simulink model "simulink_mecha_base"  (R2016b)
settings: Solver=VariableStepAuto  StartTime=0.0  StopTime=50  RelTol=1e-3
libraries: simulink x1
settings Model: Creator=Utente  LastModifiedBy=Utente

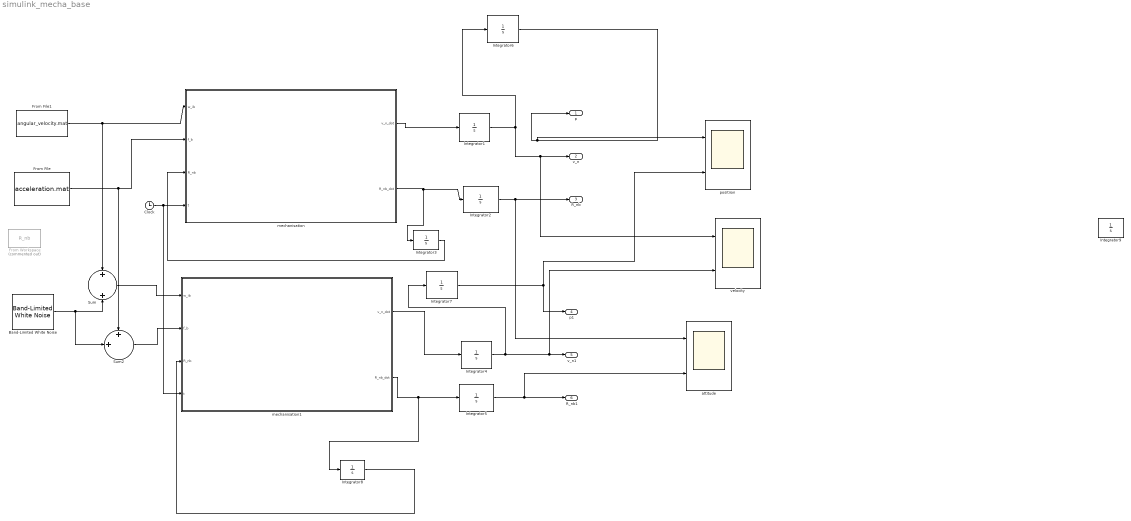
== system simulink_mecha_base ==
  Band-Limited White Noise : simulink/Sources/Band-Limited White Noise  Cov=[100 100 100]  Ts=0.1  seed=[23341]  VectorParams1D=off
  Clock : Clock
  From Workspace : FromWorkspace  Commented=on  VariableName=R_nb  SampleTime=0
  From File : FromFile  FileName=acceleration.mat  SampleTime=0
  From File1 : FromFile  FileName=angular_velocity.mat  SampleTime=0
  Integrator{1..9} (9 alike) : Integrator
  Sum : Sum  Inputs=+|+
  Sum2 : Sum  Inputs=++|
  attitude : Scope  NumInputPorts=2
  mechanisation : MATLAB Function  TreatAsAtomicUnit=on
  mechanisation1 : MATLAB Function  TreatAsAtomicUnit=on
  positiion : Scope  NumInputPorts=2
  velocity : Scope  NumInputPorts=2
  " p" : Outport
  " v_n" : Outport  Port=2
  " R_nb" : Outport  Port=3
  " p1" : Outport  Port=4
  " v_n1" : Outport  Port=5
  " R_nb1" : Outport  Port=6
  wires:
  mechanisation/1(v_n_dot) -> Integrator1/1
  Integrator1/1 -> velocity/1, " v_n"/1, Integrator6/1
  Integrator2/1 -> attitude/1, " R_nb"/1
  mechanisation1/1(v_n_dot) -> Integrator4/1
  Integrator7/1 -> " p1"/1, positiion/2
  Integrator4/1 -> Integrator7/1, velocity/2, " v_n1"/1
  Integrator5/1 -> attitude/2, " R_nb1"/1
  From File/1 -> mechanisation/2(f_b), Sum2/1
  From File1/1 -> Sum/1, mechanisation/1(w_ib)
  Band-Limited White Noise/1 -> Sum2/2, Sum/2
  Sum/1 -> mechanisation1/1(w_ib)
  Sum2/1 -> mechanisation1/2(f_b)
  Integrator6/1 -> " p"/1, positiion/1
  mechanisation/2(R_nb_dot) -> Integrator3/1, Integrator2/1
  Integrator3/1 -> mechanisation/3(R_nb)
  Clock/1 -> mechanisation1/4(t), mechanisation/4(t)
  Integrator8/1 -> mechanisation1/3(R_nb)
  mechanisation1/2(R_nb_dot) -> Integrator8/1, Integrator5/1

== matlab function simulink_mecha_base/mechanisation1 ==
  data: w_ib input; f_b input; v_n_dot output; R_nb_dot output; R_nb input; t input
function [v_n_dot, R_nb_dot] = mechanisation(w_ib, f_b, R_nb, t)



g_n = [0 0 1]';

% w_ib = size(3,1);

if t == 0
    v_n_dot = zeros(3,1);
    R_nb_dot = zeros(3,3);
    R_nb = eye(3);
end

% mechanisation

Skew = zeros(3,3);
Skew(1,2) = -w_ib(3);
Skew(2,1) = w_ib(3);
Skew(1,3) = w_ib(2);
Skew(3,1) = -w_ib(2);
Skew(2,3) = -w_ib(1);
Skew(3,2) = w_ib(1);


%p_dot = v_n;
v_n_dot = R_nb * f_b + g_n;
R_nb_dot = R_nb * Skew;

== matlab function simulink_mecha_base/mechanisation ==
  data: w_ib input; f_b input; v_n_dot output; R_nb_dot output; R_nb input; t input
function [v_n_dot, R_nb_dot] = mechanisation(w_ib, f_b, R_nb, t)



g_n = [0 0 1]';

% w_ib = size(3,1);

if t == 0
    v_n_dot = zeros(3,1);
    R_nb_dot = zeros(3,3);
    R_nb = eye(3);
end

% mechanisation

Skew = zeros(3,3);
Skew(1,2) = -w_ib(3);
Skew(2,1) = w_ib(3);
Skew(1,3) = w_ib(2);
Skew(3,1) = -w_ib(2);
Skew(2,3) = -w_ib(1);
Skew(3,2) = w_ib(1);


%p_dot = v_n;
v_n_dot = R_nb * f_b + g_n;
R_nb_dot = R_nb * Skew;
